simulink subsystem "PvtSubSys_PLAN_DPC"  (R2020b)
settings: Solver=VariableStepAuto  StartTime=0.0  StopTime=10.0  RelTol=1e-3
undefined symbols (not defined in the file or in its folder): P_Global_DxvFrontBumper_m, P_Global_DxvRearBumper_m, P_PLAN_DPC_BrkPointDxFactorF1, P_PLAN_DPC_BrkPointDxFactorF2, P_PLAN_DPC_BrkPointDxFactorF3, P_PLAN_DPC_BrkPointDxFactorF4, P_PLAN_DPC_BrkPointDxFactorR1, P_PLAN_DPC_BrkPointDxFactorR2, P_PLAN_DPC_BrkPointDxFactorR3, P_PLAN_DPC_BrkPointDxFactorR4, P_PLAN_DPC_danqianleida_kaiguan, P_PLAN_DPC_danqianleida_maxDx, P_PLAN_DPC_danqianleida_minDx, P_PLAN_DPC_FrontObj_DX_00, P_PLAN_DPC_FrontObj_DX_03, P_PLAN_DPC_FrontObj_DX_08, P_PLAN_DPC_FrontObj_DX_1, P_PLAN_DPC_HearObj_DX_00, P_PLAN_DPC_HearObj_DX_03, P_PLAN_DPC_HearObj_DX_08, P_PLAN_DPC_HearObj_DX_11, P_PLAN_DPC_HWALineRearA2Factor, P_PLAN_DPC_HWALineRearA3Factor, P_PLAN_DPC_ObjAxLPalpha, P_PLAN_DPC_ObjDxLPalpha, P_PLAN_DPC_ObjDyLPalpha, P_PLAN_DPC_ObjVxLPalpha, P_PLAN_DPC_xiangduisudu_kmh
libraries: simulink x22
(part 3 of 3)

== matlab function PvtSubSys_PLAN_DPC/DPCLock/BufRelease1 ==
  data: LaneChange input; DxvFrontBumper_m input; DxvRearBumper_m input; DPCLe input; DPCRi input; LostBufID input; LostBufRemoveMark output uint8; LostBufDx input; LostBufDy input; LostBufVx input; LostBufDPCLe input; LostBufDPCRi input; LostBufLostAge input; ObjID input; ObjDx input; ObjDy input; ObjVx input; LostBufBreakLockObjID output; LostBufBreakLockCond output; ToleranceBoxFront output; ToleranceBoxRear output; ToleranceBoxLeft output; ToleranceBoxRight output; Obj_Fus_Type input
function [LostBufRemoveMark,LostBufBreakLockObjID,LostBufBreakLockCond,ToleranceBoxFront,ToleranceBoxRear,ToleranceBoxLeft,ToleranceBoxRight]  = LostBufOut(LaneChange, DxvFrontBumper_m,DxvRearBumper_m,DPCLe,DPCRi,LostBufID,LostBufDx,LostBufDy,LostBufVx,LostBufDPCLe,LostBufDPCRi,LostBufLostAge,ObjID,ObjDx, ObjDy, ObjVx, Obj_Fus_Type)

LostBufRemoveMark=uint8(zeros(11,1));%从缓存中移除标志位
LostBufBreakLockObjID=uint8(zeros(11,1));
LostBufBreakLockCond=uint8(zeros(11,1));
ToleranceBoxFront=single(zeros(11,1));
ToleranceBoxRear=single(zeros(11,1));
ToleranceBoxLeft=single(zeros(11,1));
ToleranceBoxRight=single(zeros(11,1));

RadarUnstableZoneX=single(7);

VehCenterX=0.5*(DxvFrontBumper_m-DxvRearBumper_m);
%
for ObjIndex1 =1:11
    if LostBufID(ObjIndex1)~=uint8(0)
        MaxLocktime=max(LostBufDPCLe(ObjIndex1),LostBufDPCRi(ObjIndex1))*8;
        if  LostBufLostAge(ObjIndex1)*0.02 > MaxLocktime %如果超过锁止时间则强制释放
            LostBufRemoveMark(ObjIndex1)=uint8(1);
            LostBufBreakLockCond(ObjIndex1)=uint8(1);
            continue;
        end
        %后续可能需要根据不同位置调整公差带
        if LostBufVx(ObjIndex1)>=0
            ToleranceBoxFrontOffset=3+max(0.02*LostBufLostAge(ObjIndex1),0);%每隔1s多加一米
            ToleranceBoxRearOffset=single(3)+max(0.02*min(LostBufLostAge(ObjIndex1),100)*LostBufVx(ObjIndex1),0);%前1秒不动
            ToleranceBoxLeftOffset=single(1.8)+min(0.02*LostBufLostAge(ObjIndex1),0.8);
            ToleranceBoxRightOffset=single(1.8)+min(0.02*LostBufLostAge(ObjIndex1),0.8);
        else
            ToleranceBoxFrontOffset=single(3)+max(0.02*min(LostBufLostAge(ObjIndex1),100)*LostBufVx(ObjIndex1),0);%前1秒
            ToleranceBoxRearOffset=3+max(0.02*LostBufLostAge(ObjIndex1),0);%每隔1s加一米
            ToleranceBoxLeftOffset=single(1.8)+min(0.02*LostBufLostAge(ObjIndex1),0.8);
            ToleranceBoxRightOffset=single(1.8)+min(0.02*LostBufLostAge(ObjIndex1),0.8);
        end
        
        PreObjDx = LostBufVx(ObjIndex1)*0.02*LostBufLostAge(ObjIndex1)+LostBufDx(ObjIndex1);
        ToleranceBoxFront(ObjIndex1)=PreObjDx+ToleranceBoxFrontOffset;
        ToleranceBoxRear(ObjIndex1)=PreObjDx-ToleranceBoxRearOffset;
        ToleranceBoxLeft(ObjIndex1)=LostBufDy(ObjIndex1)+ToleranceBoxLeftOffset;
        ToleranceBoxRight(ObjIndex1)=LostBufDy(ObjIndex1)-ToleranceBoxRightOffset;
        
        %雷达不稳定区域的处理
        if ToleranceBoxFront(ObjIndex1)>VehCenterX && ToleranceBoxFront(ObjIndex1)<(DxvFrontBumper_m+RadarUnstableZoneX)
            ToleranceBoxFront(ObjIndex1)=(DxvFrontBumper_m+RadarUnstableZoneX);
        end
        if ToleranceBoxRear(ObjIndex1)>VehCenterX && ToleranceBoxRear(ObjIndex1)<(DxvFrontBumper_m+RadarUnstableZoneX)
            ToleranceBoxRear(ObjIndex1)=VehCenterX;
        end  
        if ToleranceBoxFront(ObjIndex1)>-(DxvRearBumper_m+RadarUnstableZoneX) && ToleranceBoxFront(ObjIndex1)<VehCenterX
            ToleranceBoxFront(ObjIndex1)=VehCenterX;
        end
        if ToleranceBoxRear(ObjIndex1)>-(DxvRearBumper_m+RadarUnstableZoneX) && ToleranceBoxRear(ObjIndex1)<VehCenterX
            ToleranceBoxRear(ObjIndex1)=-(DxvRearBumper_m+RadarUnstableZoneX);
        end
            
        for ObjIndex2 =1:11 
            %如果20帧内重新找到ID则停止锁定
            if ObjID(ObjIndex2)==LostBufID(ObjIndex1) && LostBufLostAge(ObjIndex1)<=20 && Obj_Fus_Type(ObjIndex2) ~= 0
                LostBufRemoveMark(ObjIndex1)=uint8(1);
                LostBufBreakLockObjID(ObjIndex1)=ObjID(ObjIndex2);
                LostBufBreakLockCond(ObjIndex1)=uint8(2);
                break;
            end
            %在预测位置存在一个目标则停止锁定
            if ObjID(ObjIndex2)~= uint8(0) ...
                    && ObjDx(ObjIndex2) <= ToleranceBoxFront(ObjIndex1)...
                    && ObjDx(ObjIndex2) >= ToleranceBoxRear(ObjIndex1)...
                    && ObjDy(ObjIndex2) <= ToleranceBoxLeft(ObjIndex1)...
                    && ObjDy(ObjIndex2) >= ToleranceBoxRight(ObjIndex1) &&  Obj_Fus_Type(ObjIndex2) ~= 0
                LostBufRemoveMark(ObjIndex1)=uint8(1);
                LostBufBreakLockObjID(ObjIndex1)=ObjID(ObjIndex2);
                LostBufBreakLockCond(ObjIndex1)=uint8(3);
                break;
            end
        end
    end

if LaneChange
    LostBufRemoveMark=uint8(ones(11,1));
    LostBufBreakLockCond=uint8(4*ones(11,1));
end
end

== matlab function PvtSubSys_PLAN_DPC/DPCLock/LPF/MATLAB Function ==
  data: Alpha input; ID input; IDK1 input; signal input; result output; resultK1 input single
function result  = LowPassFilter(Alpha,ID,IDK1,signal,resultK1)
result=single(zeros(11,1));
for i=1:11
[IDSurvive,IDoldIndex]=ismember(ID(i),IDK1);
if ID(i)~=uint8(0) && IDSurvive
    result(i) = Alpha*(signal(i) - resultK1(IDoldIndex)) + resultK1(IDoldIndex);
else
    result(i)=signal(i);
end
end

== matlab function PvtSubSys_PLAN_DPC/DPCLock/LPF/MATLAB Function1 ==
  data: Alpha input; ID input; IDK1 input; signal input; result output; resultK1 input single
function result  = LowPassFilter(Alpha,ID,IDK1,signal,resultK1)
result=single(zeros(11,1));
for i=1:11
[IDSurvive,IDoldIndex]=ismember(ID(i),IDK1);
if ID(i)~=uint8(0) && IDSurvive
    result(i) = Alpha*(signal(i) - resultK1(IDoldIndex)) + resultK1(IDoldIndex);
else
    result(i)=signal(i);
end
end

== matlab function PvtSubSys_PLAN_DPC/DPCLock/LPF/MATLAB Function2 ==
  data: Alpha input; ID input; IDK1 input; signal input; result output; resultK1 input single
function result  = LowPassFilter(Alpha,ID,IDK1,signal,resultK1)
result=single(zeros(11,1));
for i=1:11
[IDSurvive,IDoldIndex]=ismember(ID(i),IDK1);
if ID(i)~=uint8(0) && IDSurvive
    result(i) = Alpha*(signal(i) - resultK1(IDoldIndex)) + resultK1(IDoldIndex);
else
    result(i)=signal(i);
end
end

== matlab function PvtSubSys_PLAN_DPC/DPCLock/LPF/MATLAB Function3 ==
  data: LineValid input; LineC3 input; SLObjDy output; LineC2 input; LineC1 input; LineC0 input; LineRange input; ObjDy input; ObjDx input
function SLObjDy=SLdyclc(LineValid,LineC3,LineC2,LineC1,LineC0,LineRange,ObjDy,ObjDx)
SLObjDy=single(zeros(11,1));
for i=1:11
    if  ObjDx(i)>0
        LineC3Factor = single(0);
        LineC2Factor = Interp4(0, 1, LineRange, 1, LineRange+20, 0.7, LineRange+40, 0, ObjDx(i));
        dLineDy = (LineC3Factor * LineC3 * ObjDx(i) * ObjDx(i) * ObjDx(i)) + (LineC2Factor * LineC2 * ObjDx(i) * ObjDx(i)) + (LineC1 * ObjDx(i)) + LineC0;
        SLObjDy(i) = ObjDy(i)-dLineDy;
    else 
        LineC3Factor = single(0);
        LineC2Factor = single(0.2);
        dLineDy = ((LineC3Factor * LineC3 * ObjDx(i) * ObjDx(i) * ObjDx(i)) + (LineC2Factor * LineC2 * ObjDx(i) * ObjDx(i)) + (LineC1 * ObjDx(i)) + LineC0);
        SLObjDy(i) = ObjDy(i)-dLineDy;
    end
end
end
function Out = Interp4(x1,z1,x2,z2,x3,z3,x4,z4,In)  %线性插值
if In<=x1
    Out = single(z1);
elseif (In>x1)&&(In<=x2)
    Out = single(z1+ (In-x1)*(z2-z1)/(x2-x1));
elseif (In>x2)&&(In<=x3)
    Out = single(z2+ (In-x2)*(z3-z2)/(x3-x2));
elseif (In>x3)&&(In<=x4)
    Out = single(z3+ (In-x3)*(z4-z3)/(x4-x3));
else
    Out = single(z4);
end
end

== matlab function PvtSubSys_PLAN_DPC/DPCLock/Lock ==
  data: bufferoverflow output; LostBufRemoveMark input; ObjDPCleK1 input; ObjDPCRiK1 input; ObjID input; ObjIDK1 input; ObjDxK1 input; ObjDyK1 input; ObjVxK1 input; LostBufIDK1 input; LostBufDxK1 input; LostBufDyK1 input; LostBufVxK1 input; LostBufDPCLeK1 input; LostBufDPCRiK1 input; LostBufLostAgeK1 input; LostBufID output uint8; LostBufDx output single; LostBufDy output single; LostBufVx output single; LostBufDPCLe output single; LostBufDPCRi output; LostBufLostAge output single
function [bufferoverflow,LostBufID,LostBufDx,LostBufDy,LostBufVx,LostBufDPCLe,LostBufDPCRi,LostBufLostAge] = TimeCalc(LostBufRemoveMark,ObjDPCleK1,ObjDPCRiK1,ObjID,ObjIDK1,ObjDxK1,ObjDyK1,ObjVxK1,LostBufIDK1,LostBufDxK1,LostBufDyK1,LostBufVxK1,LostBufDPCLeK1,LostBufDPCRiK1,LostBufLostAgeK1)

LostBufID=LostBufIDK1;
LostBufDx=LostBufDxK1;
LostBufDy=LostBufDyK1;
LostBufVx=LostBufVxK1;
LostBufDPCLe=LostBufDPCLeK1;
LostBufDPCRi=LostBufDPCRiK1;
LostBufLostAge=LostBufLostAgeK1;
bufferoverflow=false;

%删除被标记需要释放的元素  //释放目标直接赋予0//
for ObjIndex1=1:11%11个目标
    if LostBufRemoveMark(ObjIndex1)~=uint8(0) %不等于0 说明是1//
        LostBufID(ObjIndex1)=uint8(0);
        LostBufDx(ObjIndex1)=single(0);
        LostBufDy(ObjIndex1)=single(0);
        LostBufVx(ObjIndex1)=single(0);
        LostBufDPCLe(ObjIndex1)=single(0);
        LostBufDPCRi(ObjIndex1)=single(0);
        LostBufLostAge(ObjIndex1)=single(0);
    end
end

% 寻找是否有ID丢失并存入buf
for ObjIndex1=1:11
    if ObjIDK1(ObjIndex1)~=0 %上一周期ID不等于0//
        %寻找过程
        findID=false;
        for ObjIndex2 =1:11
            if ObjID(ObjIndex2)==ObjIDK1(ObjIndex1) %当前时刻的id == 上一时刻的id////
                findID=true;
                break;
            end
        end
        %储存过程
        if ~findID %findID没有找到  那就走这个if 这是丢了//
            MaxLostAge=single(0);
            findbufposition=false;
            bufferoverflow=false;
            oldestbufIndex=11;
            for ObjIndex2 =1:11
                if LostBufLostAge(ObjIndex2)>MaxLostAge %LostBufLostAge这是啥意思//
                    MaxLostAge=LostBufLostAge(ObjIndex2);
                    oldestbufIndex=ObjIndex2;
                end
                if LostBufID(ObjIndex2)==0 %缓存未被使用   %这是什么意思///
                    LostBufID(ObjIndex2)=ObjIDK1(ObjIndex1);
                    LostBufDx(ObjIndex2)=ObjDxK1(ObjIndex1);
                    LostBufDy(ObjIndex2)=ObjDyK1(ObjIndex1);
                    LostBufVx(ObjIndex2)=ObjVxK1(ObjIndex1);
                    LostBufDPCLe(ObjIndex2)=ObjDPCleK1(ObjIndex1);
                    LostBufDPCRi(ObjIndex2)=ObjDPCRiK1(ObjIndex1);
                    findbufposition=true;
                    break;
                end
            end
            if ~findbufposition
                LostBufID(oldestbufIndex)=ObjIDK1(ObjIndex1);
                LostBufDx(oldestbufIndex)=ObjDxK1(ObjIndex1);
                LostBufDy(oldestbufIndex)=ObjDyK1(ObjIndex1);
                LostBufVx(oldestbufIndex)=ObjVxK1(ObjIndex1);
                LostBufDPCLe(oldestbufIndex)=ObjDPCleK1(ObjIndex1);
                LostBufDPCRi(oldestbufIndex)=ObjDPCRiK1(ObjIndex1);
                bufferoverflow=true;
            end
            
        end
    end
end

%计算丢失的周期，从1开始
for ObjIndex1 =1:11
    if LostBufID(ObjIndex1)~=uint8(0)
        LostBufLostAge(ObjIndex1)=min(LostBufLostAge(ObjIndex1)+1,500);%LostBufLostAge记录目标丢的时间///
    end
end

%坐标旋转
% for ObjIndex1 =1:11
%     LostBufDx(ObjIndex1) = (LostBufDx(ObjIndex1)-EgoDDeltaX)*EgoCosOfPsi + (LostBufDy(ObjIndex1)-EgoDDeltaY)*EgoSinOfPsi;
%     LostBufDy(ObjIndex1) = -(LostBufDx(ObjIndex1)-EgoDDeltaX)*EgoSinOfPsi + (LostBufDy(ObjIndex1)-EgoDDeltaY)*EgoCosOfPsi;
% end
end

== matlab function PvtSubSys_PLAN_DPC/DPCLock/Release ==
  data: DPCLe input; DPCRi input; LostBufID input; LostBufRemoveMark output uint8; LostBufDx input; LostBufDy input; LostBufVx input; LostBufDPCLe input; LostBufDPCRi input; LostBufLostAge input; ObjID input; ObjDx input; ObjDy input; ObjVx input
function LostBufRemoveMark  = fcn(DPCLe,DPCRi,LostBufID,LostBufDx,LostBufDy,LostBufVx,LostBufDPCLe,LostBufDPCRi,LostBufLostAge,ObjID,ObjDx, ObjDy, ObjVx )

LostBufRemoveMark=uint8(zeros(11,1));
FrontLine1=8;%前向角雷达属性不稳定限制线
RearLine1=-6;%后向角雷达属性不稳定限制线
PreDxOffSet=5;%允许的预测误差

for ObjIndex1 =1:11 %如果超过锁止时间则强制释放
    if LostBufID(ObjIndex1)~=0
        Locktime=max(LostBufDPCLe(ObjIndex1),LostBufDPCRi(ObjIndex1))*10;
        if  LostBufLostAge(ObjIndex1)>Locktime
            LostBufRemoveMark(ObjIndex1)=uint8(1);
        end
    end
end
for ObjIndex1 =1:11
    if LostBufID(ObjIndex1)~=0
        for ObjIndex2 =1:11 %如果十个周期内重新找到ID则停止锁定
            PreObjDx = LostBufVx(ObjIndex1)*LostBufLostAge(ObjIndex1)+LostBufDx(ObjIndex1);
            if ObjID(ObjIndex2)==LostBufID(ObjIndex1) && LostBufLostAge(ObjIndex1)<=10
                LostBufRemoveMark(ObjIndex1)=uint8(1);
                break;
            end
            if LostBufDy(ObjIndex1) > 0 && abs(ObjDx(ObjIndex2)-PreObjDx) < PreDxOffSet && ObjDy(ObjIndex2) > 0  && ObjID(ObjIndex2)~=0 %分两边 如果预测位置有目标则解除锁定
                LostBufRemoveMark(ObjIndex1)=uint8(1);
                break;
            end
            if LostBufDy(ObjIndex1) <= 0 && abs(ObjDx(ObjIndex2)-PreObjDx) < PreDxOffSet && ObjDy(ObjIndex2) <= 0  && ObjID(ObjIndex2)~=0 %分两边 如果预测位置有目标则解除锁定
                LostBufRemoveMark(ObjIndex1)=uint8(1);
                break;
            end
            if PreObjDx<FrontLine1 && PreObjDx>RearLine1 && LostBufDy(ObjIndex1) > 0 && ObjDx(ObjIndex2)<FrontLine1 && ObjDx(ObjIndex2)>RearLine1 && ObjDy(ObjIndex2) > 0 && ObjID(ObjIndex2)~=0  %分两边 前后雷达不可信属性区域内消失的目标,特殊处理一下
                LostBufRemoveMark(ObjIndex1)=uint8(1);
                break;
            end
            if PreObjDx<FrontLine1 && PreObjDx>RearLine1 && LostBufDy(ObjIndex1) <= 0 && ObjDx(ObjIndex2)<FrontLine1 && ObjDx(ObjIndex2)>RearLine1 && ObjDy(ObjIndex2) <= 0 && ObjID(ObjIndex2)~=0  %分两边 前后雷达不可信属性区域内消失的目标,特殊处理一下
                LostBufRemoveMark(ObjIndex1)=uint8(1);
                break;             
            end
            if LostBufDx(ObjIndex1)<FrontLine1 && LostBufDx(ObjIndex1)>RearLine1 && LostBufDy(ObjIndex1) > 0 && ObjDx(ObjIndex2)<FrontLine1 && ObjDx(ObjIndex2)>RearLine1 && ObjDy(ObjIndex2) > 0 && ObjID(ObjIndex2)~=0  %分两边 预测会进入该不可信区域的目标特殊处理一下
                LostBufRemoveMark(ObjIndex1)=uint8(1);
                break;
            end
            if LostBufDx(ObjIndex1)<FrontLine1 && LostBufDx(ObjIndex1)>RearLine1 && LostBufDy(ObjIndex1) <= 0 && ObjDx(ObjIndex2)<FrontLine1 && ObjDx(ObjIndex2)>RearLine1 && ObjDy(ObjIndex2) <= 0 && ObjID(ObjIndex2)~=0  %分两边 预测会进入该不可信区域的目标特殊处理一下
                LostBufRemoveMark(ObjIndex1)=uint8(1);
                break;             
            end
        end
    end
end

== matlab function PvtSubSys_PLAN_DPC/DPCLock/Release1 ==
  data: DPCLe input; DPCRi input; LostBufID input; LostBufRemoveMark output uint8; LostBufDx input; LostBufDy input; LostBufVx input; LostBufDPCLe input; LostBufDPCRi input; LostBufLostAge input; ObjID input; ObjDx input; ObjDy input; ObjVx input
function LostBufRemoveMark  = fcn(DPCLe,DPCRi,LostBufID,LostBufDx,LostBufDy,LostBufVx,LostBufDPCLe,LostBufDPCRi,LostBufLostAge,ObjID,ObjDx, ObjDy, ObjVx )

LostBufRemoveMark=uint8(zeros(11,1));
FrontLine1=8;%前向角雷达属性不稳定限制线
RearLine1=-6;%后向角雷达属性不稳定限制线
PreDxOffSet=5;%允许的预测误差

for ObjIndex1 =1:11 %如果超过锁止时间则强制释放
    if LostBufID(ObjIndex1)~=0
        Locktime=max(LostBufDPCLe(ObjIndex1),LostBufDPCRi(ObjIndex1))*10;
        if  LostBufLostAge(ObjIndex1)>Locktime
            LostBufRemoveMark(ObjIndex1)=uint8(1);
        end
    end
end
for ObjIndex1 =1:11 
    if LostBufID(ObjIndex1)~=0
        PreObjDx = LostBufVx(ObjIndex1)*LostBufLostAge(ObjIndex1)+LostBufDx(ObjIndex1);
        for ObjIndex2 =1:11 %如果十个周期内重新找到ID则停止锁定
            if ObjID(ObjIndex2)==LostBufID(ObjIndex1) && LostBufLostAge(ObjIndex1)<=10
                LostBufRemoveMark(ObjIndex1)=uint8(1);
                break;
            end
        end
        if LostBufDy(ObjIndex1) > 0 %分两边 如果预测位置有目标则解除锁定
            for ObjIndex2 =1:11
                if abs(ObjDx(ObjIndex2)-PreObjDx) < PreDxOffSet && ObjDy(ObjIndex2) > 0  && ObjID(ObjIndex2)~=0
                    LostBufRemoveMark(ObjIndex1)=uint8(1);
                    break;
                end
            end
        end
        if LostBufDy(ObjIndex1) <= 0  %分两边 如果预测位置有目标则解除锁定
            for ObjIndex2 =1:11
                if abs(ObjDx(ObjIndex2)-PreObjDx) < PreDxOffSet && ObjDy(ObjIndex2) <= 0  && ObjID(ObjIndex2)~=0
                    LostBufRemoveMark(ObjIndex1)=uint8(1);
                    break;
                end
            end
        end
        if (LostBufDx(ObjIndex1)<FrontLine1 || PreObjDx<FrontLine1) && (LostBufDx(ObjIndex1)>RearLine1 || PreObjDx>RearLine1) && LostBufDy(ObjIndex1) < 0   %分两边 前后雷达不可信属性区域内消失的目标特殊处理一下
            for ObjIndex2 =1:11
                if ObjDx(ObjIndex2)<FrontLine1 && ObjDx(ObjIndex2)>RearLine1 && ObjDy(ObjIndex2) < 0 && ObjID(ObjIndex2)~=0
                    LostBufRemoveMark(ObjIndex1)=uint8(1);
                    break;
                end
            end
        end
        if (LostBufDx(ObjIndex1)<FrontLine1 || PreObjDx<FrontLine1) && (LostBufDx(ObjIndex1)>RearLine1 || PreObjDx>RearLine1) && LostBufDy(ObjIndex1) > 0 
            for ObjIndex2 =1:11
                if ObjDx(ObjIndex2)<FrontLine1 && ObjDx(ObjIndex2)>RearLine1 && ObjDy(ObjIndex2) > 0 && ObjID(ObjIndex2)~=0
                    LostBufRemoveMark(ObjIndex1)=uint8(1);
                    break;
                end
            end
        end      
    end
end

== matlab function PvtSubSys_PLAN_DPC/DangerPlausCalc/DangerPlaus_Calculate_Radar ==
  data: ObjID input; ObjTimeAlive input; ObjDx input; ObjDxRelCal_FL output; ObjDxRelCal_FR output; ObjDxRelCal_RL output; ObjDxRelCal_RR output; ObjDy input; ObjVx input; Object_Fus_Type input; Object_MovingState input; ESSLineLA3 input; ESSLineLA2 input; ESSLineLA1 input; ESSLineLA0 input; ESSLineLRange input; ESSLineRA3 input; ESSLineRA2 input; ESSLineRA1 input; ESSLineRA0 input; ESSLineRRange input; VehicleSpd_kph input; RoadWidth input; Y_Factor_L output; Y_Factor_R output; L_Oncoming_flag output; R_Oncoming_flag output; NearestObjValid_L output boolean; NearestObjValid_R output boolean; NearestObjSpeed_L output; NearestObjSpeed_R output; ObjVxGnd_1 output; ObjDxRelFinal_FL_1 output; P_VSM_DPC_HWALineRearA2Factor input; P_VSM_DPC_HWALineRearA3Factor input; P_Global_DxvFrontBumper_m input; P_Global_DxvRearBumper_m input
function [ObjDxRelCal_FL,ObjDxRelCal_FR,ObjDxRelCal_RL,ObjDxRelCal_RR,Y_Factor_L,Y_Factor_R,...
    L_Oncoming_flag,R_Oncoming_flag,...
    NearestObjValid_L,NearestObjValid_R,NearestObjSpeed_L,NearestObjSpeed_R, ObjVxGnd_1, ObjDxRelFinal_FL_1] = ...
    fcn(ObjID, ObjTimeAlive, ObjDx, ObjDy, ObjVx, Object_Fus_Type, Object_MovingState,...
    ESSLineLA3, ESSLineLA2,ESSLineLA1, ESSLineLA0, ESSLineLRange,...
    ESSLineRA3, ESSLineRA2,ESSLineRA1, ESSLineRA0, ESSLineRRange,...
    VehicleSpd_kph,RoadWidth,...
    P_VSM_DPC_HWALineRearA2Factor,...
P_VSM_DPC_HWALineRearA3Factor, P_Global_DxvFrontBumper_m, P_Global_DxvRearBumper_m)

InvalidValue = single(999);
ObjTimeAliveCounter = 3;
TimeTurn = 4;
TimeReact = 3;
ObjDxRelCal_FL = zeros(11,1);
ObjDxRelCal_FR = zeros(11,1);
ObjDxRelCal_RL = zeros(11,1);
ObjDxRelCal_RR = zeros(11,1);
DeltaDistance_Y_L = zeros(11,1);
DeltaDistance_Y_R = zeros(11,1);
Y_Factor_L = zeros(11,1);
Y_Factor_R = zeros(11,1);
L_Oncoming = zeros(11,1);
R_Oncoming = zeros(11,1);
VehicleSpd_ms = VehicleSpd_kph / 3.6;

TimePredict_L = (abs(ESSLineLA0) / RoadWidth * TimeTurn) + TimeReact;
TimePredict_R = (abs(ESSLineRA0) / RoadWidth * TimeTurn) + TimeReact;

NearestObjValid_L = false;
NearestObjDx_L = InvalidValue;
NearestObjSpeed_L = InvalidValue;
NearestObjValid_R = false;
NearestObjDx_R = InvalidValue;
NearestObjSpeed_R = InvalidValue;

ObjVxGnd_1 = single(0);
ObjDxRelFinal_FL_1 = single(0);

for i = 1:11
    if (ObjID(i) > 0)...
            && (ObjTimeAlive(i) > ObjTimeAliveCounter)
        ObjVxGnd = ObjVx(i) + VehicleSpd_ms;
        if i == 1   %%%TEST
            ObjVxGnd_1 = ObjVxGnd;
        end
        if ObjDx(i) >= 0   %Front
            ObjDxRelCal_RL(i) = - InvalidValue;
            ObjDxRelCal_RR(i) = - InvalidValue;
            %%%X Calculate%%%
            ObjDxRelInitial_Front = ObjDx(i) - P_Global_DxvFrontBumper_m;
            ObjDxRelFinal_FL = ObjDxRelInitial_Front + (ObjVxGnd * TimePredict_L) - (VehicleSpd_ms * TimePredict_L);
            if i == 1   %%%TEST
                ObjDxRelFinal_FL_1 = ObjDxRelFinal_FL;
            end
            ObjDxRelFinal_FR = ObjDxRelInitial_Front + (ObjVxGnd * TimePredict_R) - (VehicleSpd_ms * TimePredict_R);
            if (ObjDxRelInitial_Front*ObjDxRelFinal_FL)<0   %Very Dangerous
                ObjDxRelCal_FL(i) = 0;
            else
                ObjDxRelCal_FL(i) = min(ObjDxRelInitial_Front,ObjDxRelFinal_FL);
            end
            if (ObjDxRelInitial_Front*ObjDxRelFinal_FR)<0
                ObjDxRelCal_FR(i) = 0;
            else
                ObjDxRelCal_FR(i) = min(ObjDxRelInitial_Front,ObjDxRelFinal_FR);
            end
            %%%Y Calculate%%%
            P_HWALineLFrontA3Factor = single(0);
            P_HWALineRFrontA3Factor = single(0);
            P_HWALineLFrontA2Factor = Interpol(0, 1, ESSLineLRange, 1, ESSLineLRange+20, 0.7, ESSLineLRange+40, 0, ObjDx(i));
            P_HWALineRFrontA2Factor = Interpol(0, 1, ESSLineRRange, 1, ESSLineRRange+20, 0.7, ESSLineRRange+40, 0, ObjDx(i));
            Y_L = (P_HWALineLFrontA3Factor * ESSLineLA3 * ObjDx(i) * ObjDx(i) * ObjDx(i)) + (P_HWALineLFrontA2Factor * ESSLineLA2 * ObjDx(i) * ObjDx(i)) + (ESSLineLA1 * ObjDx(i)) + ESSLineLA0;
            Y_R = (P_HWALineRFrontA3Factor * ESSLineRA3 * ObjDx(i) * ObjDx(i) * ObjDx(i)) + (P_HWALineRFrontA2Factor * ESSLineRA2 * ObjDx(i) * ObjDx(i)) + (ESSLineRA1 * ObjDx(i)) + ESSLineRA0;
            %%%SD%%%
            DeltaDistance_Y_L(i) = abs(ObjDy(i) - Y_L);
            DeltaDistance_Y_R(i) = abs(ObjDy(i) - Y_R);
            %%%Feature Of Nearest Obj Of Next Lane%%%
            if (ObjDy(i) >= (Y_L - (RoadWidth / 2))) && (ObjDy(i) <= (Y_L + (RoadWidth / 2))) && (ObjDx(i) <= NearestObjDx_L)
                NearestObjValid_L = true;
                NearestObjDx_L = ObjDx(i);
                NearestObjSpeed_L = ObjVxGnd;
                if NearestObjSpeed_L < 0
                    L_Oncoming(i) = 1;
                else
                    L_Oncoming(i) = 0;
                end
            elseif (ObjDy(i) >= (Y_R - (RoadWidth / 2))) && (ObjDy(i) <= (Y_R + (RoadWidth / 2))) && (ObjDx(i) <= NearestObjDx_R)
                NearestObjValid_R = true;
                NearestObjDx_R = ObjDx(i);
                NearestObjSpeed_R = ObjVxGnd;
                if NearestObjSpeed_R < 0
                    R_Oncoming(i) = 1;
                else
                    R_Oncoming(i) = 0;
                end
            end
        else   %Rear
            ObjDxRelCal_FL(i) = InvalidValue;
            ObjDxRelCal_FR(i) = InvalidValue;
            %%%X Calculate%%%
            ObjDxRelInitial_Rear = ObjDx(i) + P_Global_DxvRearBumper_m;
            ObjDxRelFinal_RL = ObjDxRelInitial_Rear + (ObjVxGnd * TimePredict_L) - (VehicleSpd_ms * TimePredict_L);
            ObjDxRelFinal_RR = ObjDxRelInitial_Rear + (ObjVxGnd * TimePredict_R) - (VehicleSpd_ms * TimePredict_R);
            if (ObjDxRelInitial_Rear*ObjDxRelFinal_RL)<0
                ObjDxRelCal_RL(i) = 0;
            else
                ObjDxRelCal_RL(i) = max(ObjDxRelInitial_Rear,ObjDxRelFinal_RL);
            end
            
            if (ObjDxRelInitial_Rear*ObjDxRelFinal_RR)<0
                ObjDxRelCal_RR(i) = 0;
            else
                ObjDxRelCal_RR(i) = max(ObjDxRelInitial_Rear,ObjDxRelFinal_RR);
            end
            %%%Y Calculate%%%
            Y_L = (P_VSM_DPC_HWALineRearA3Factor * ESSLineLA3 * ObjDx(i) * ObjDx(i) * ObjDx(i)) + (P_VSM_DPC_HWALineRearA2Factor * ESSLineLA2 * ObjDx(i) * ObjDx(i)) + (ESSLineLA1 * ObjDx(i)) + ESSLineLA0;
            Y_R = (P_VSM_DPC_HWALineRearA3Factor * ESSLineRA3 * ObjDx(i) * ObjDx(i) * ObjDx(i)) + (P_VSM_DPC_HWALineRearA2Factor * ESSLineRA2 * ObjDx(i) * ObjDx(i)) + (ESSLineRA1 * ObjDx(i)) + ESSLineRA0;
            %%%SD%%%
            DeltaDistance_Y_L(i) = abs(ObjDy(i) - Y_L);
            DeltaDistance_Y_R(i) = abs(ObjDy(i) - Y_R);
        end
    else
        ObjDxRelCal_FL(i) = InvalidValue;
        ObjDxRelCal_FR(i) = InvalidValue;
        ObjDxRelCal_RL(i) = - InvalidValue;
        ObjDxRelCal_RR(i) = - InvalidValue;
        DeltaDistance_Y_L(i) = InvalidValue;
        DeltaDistance_Y_R(i) = InvalidValue;
    end
    if (Object_Fus_Type(i) == 0x2) && (Object_MovingState(i) == 0x3)   %F&&Stationary
        Y_Factor_L(i) = Interpol(0, 1, 0.3*RoadWidth, 1, 0.6*RoadWidth, 0, 0.6*RoadWidth+1, 0, DeltaDistance_Y_L(i));
        Y_Factor_R(i) = Interpol(0, 1, 0.3*RoadWidth, 1, 0.6*RoadWidth, 0, 0.6*RoadWidth+1, 0, DeltaDistance_Y_R(i));
    else
        Y_Factor_L(i) = Interpol(0, 1, 0.5*RoadWidth, 1, 0.5*RoadWidth+1, 0, 0.5*RoadWidth+2, 0, DeltaDistance_Y_L(i));
        Y_Factor_R(i) = Interpol(0, 1, 0.5*RoadWidth, 1, 0.5*RoadWidth+1, 0, 0.5*RoadWidth+2, 0, DeltaDistance_Y_R(i));
    end
    L_Oncoming_flag = ismember(1,L_Oncoming);
    R_Oncoming_flag = ismember(1,R_Oncoming);
end

function Out = Interpol(x1,z1,x2,z2,x3,z3,x4,z4,In)
if In<=x1
    Out = single(z1);
elseif (In>x1)&&(In<=x2)
    Out = single(z1+ (In-x1)*(z2-z1)/(x2-x1));
elseif (In>x2)&&(In<=x3)
    Out = single(z2+ (In-x2)*(z3-z2)/(x3-x2));
elseif (In>x3)&&(In<=x4)
    Out = single(z3+ (In-x3)*(z4-z3)/(x4-x3));
else
    Out = single(z4);
end

== matlab function PvtSubSys_PLAN_DPC/DangerPlausCalc3/DangerFactorMatrixCalc_Left ==
  data: VehSpd input; ObjValid input; ObjDx input; ObjDy input; ObjVx input; LineValid input; LineC3 input; LineC2 input; LineC1 input; LineC0 input; LineRange input; LineRearC2Factor input; LineRearC3Factor input; RoadWidth input; MaxObjNum input; obj_front_Dx output; obj_front_Vx output size=[1 11]; obj_Rear_Dx output; obj_Rear_Vx output; PreDyRel output size=[11]; Oncoming_flag output; NearestObjValid output; NearestObjDx output; NearestObjSpeed output; Rear_NearesObjValid output; Rear_NearestObjDx output; Rear_NearestObjSpeed output
function [obj_front_Dx,obj_front_Vx,obj_Rear_Dx,obj_Rear_Vx,PreDyRel,Oncoming_flag,NearestObjValid,NearestObjDx,NearestObjSpeed,Rear_NearesObjValid,Rear_NearestObjDx,Rear_NearestObjSpeed] = ...
    fcn(VehSpd,ObjValid,ObjDx, ObjDy, ObjVx, ...
    LineValid, LineC3, LineC2,LineC1, LineC0, LineRange,...
    LineRearC2Factor,LineRearC3Factor,RoadWidth,MaxObjNum)
% #define
fInvalidValue = single(999);%无效值

%init

PreDyRel = ones(11,1).*fInvalidValue;

NearestObjValid = false;
NearestObjDx = fInvalidValue;
NearestObjSpeed = fInvalidValue;
%/////
Rear_NearesObjValid = false;
Rear_NearestObjDx = -fInvalidValue;
Rear_NearestObjSpeed = -fInvalidValue;
%/////
NearestObj_Oncoming = zeros(11,1);

DxvFrontBumper_m = single(3.8);

DxvRearBumper_m = single(0.9);
RtVehSpdms=VehSpd/3.6;





%新接口信号
Front_fInvalidValue = single(999);%无效值
Rear_fInvalidValue = single(-999);%无效值
obj_front_Dx = ones(1,11).* Front_fInvalidValue;
obj_front_Vx = single(zeros(1,11));
obj_Rear_Dx = ones(1,11).* Rear_fInvalidValue;
obj_Rear_Vx = single(zeros(1,11));



%ObjVx 单位是m/s  /////////

if LineValid ~= 0
    for i = 1:MaxObjNum
        if ObjValid(i) 
                if ObjDx(i) >= 0 %前方目标
                  obj_front_Dx(i) = ObjDx(i);%-0.2-DxvFrontBumper_m;
                  obj_front_Vx(i) = single(ObjVx(i)*3.6+0.5);%m/s转换成km/h  ////////////    
                else %后方目标
                    % dPreCollisionDist = ObjDx(i) + DxvRearBumper_m;%障碍物到车屁股的距离//负值
                  obj_Rear_Dx(i) = ObjDx(i);%-0.2+ DxvRearBumper_m;
                  obj_Rear_Vx(i) = single(ObjVx(i)*3.6+0.5);%m/s转换成km/h  //////////// 
                end
        else
            %do nothing
        end
        %计算横向相对距离和前方目标属性
        if ObjDx(i) >= 0 %前方目标
            LineC3Factor = single(0);
            LineC2Factor = Interp4(0, 1, LineRange, 1, LineRange+20, 0.7, LineRange+40, 0, ObjDx(i));
            dLineDy=(LineC3Factor * LineC3 * ObjDx(i) * ObjDx(i) * ObjDx(i)) + (LineC2Factor * LineC2 * ObjDx(i) * ObjDx(i)) + (LineC1 * ObjDx(i)) + LineC0;
            PreDyRel(i) = ObjDy(i)-dLineDy;
            %前方最近目标属性
            if (ObjDy(i) >= (dLineDy - (RoadWidth / 2))) && (ObjDy(i) <= (dLineDy + (RoadWidth / 2))) && (ObjDx(i) <= NearestObjDx)
                ObjVx_GND = RtVehSpdms + ObjVx(i);
                NearestObjValid = true;
                NearestObjDx = ObjDx(i);
                NearestObjSpeed = ObjVx_GND;
                if NearestObjSpeed < -2.5
                    NearestObj_Oncoming(i) = 1;
                    
                else
                    NearestObj_Oncoming(i) = 0;
                end
            end
        else %后方目标
            %计算横向相对距离
            LineC3Factor = LineRearC3Factor;
            LineC2Factor = LineRearC2Factor;
            dLineDy = ((LineC3Factor * LineC3 * ObjDx(i) * ObjDx(i) * ObjDx(i)) + (LineC2Factor * LineC2 * ObjDx(i) * ObjDx(i)) + (LineC1 * ObjDx(i)) + LineC0);
            PreDyRel(i) = ObjDy(i)-dLineDy;
            %后方最近目标属性
            if (ObjDy(i) >= (dLineDy - (RoadWidth / 2))) && (ObjDy(i) <= (dLineDy + (RoadWidth / 2))) && (ObjDx(i) >= Rear_NearestObjDx)
               ObjVx_GND = RtVehSpdms + ObjVx(i);
               Rear_NearesObjValid = true;
               Rear_NearestObjDx = ObjDx(i);
               Rear_NearestObjSpeed = ObjVx_GND; %绝对速度//
            end
            
        end
    end
    Oncoming_flag = ismember(1,NearestObj_Oncoming);
    
else
    PreDyRel = single(zeros(11,1));
    Oncoming_flag = false;
    NearestObjValid = false;
    Rear_NearesObjValid = false;
    obj_front_Vx = single(zeros(1,11));
    obj_Rear_Vx = single(zeros(1,11));
    obj_front_Dx = ones(1,11).* Front_fInvalidValue;
    obj_Rear_Dx = ones(1,11).* Rear_fInvalidValue;
    
end

end


function Out = Interp4(x1,z1,x2,z2,x3,z3,x4,z4,In)  %线性插值
if In<=x1
    Out = single(z1);
elseif (In>x1)&&(In<=x2)
    Out = single(z1+ (In-x1)*(z2-z1)/(x2-x1));
elseif (In>x2)&&(In<=x3)
    Out = single(z2+ (In-x2)*(z3-z2)/(x3-x2));
elseif (In>x3)&&(In<=x4)
    Out = single(z3+ (In-x3)*(z4-z3)/(x4-x3));
else
    Out = single(z4);
end
end

== matlab function PvtSubSys_PLAN_DPC/DangerPlausCalc3/DangerFactorMatrixCalc_Left1 ==
  data: VehSpd input; ObjValid input; ObjDx input; ObjDy input; ObjVx input; LineValid input; LineC3 input; LineC2 input; LineC1 input; LineC0 input; LineRange input; LineRearC2Factor input; LineRearC3Factor input; RoadWidth input; MaxObjNum input; obj_front_Dx output; obj_front_Vx output size=[1 11]; obj_Rear_Dx output; obj_Rear_Vx output; PreDyRel output size=[11]; Oncoming_flag output; NearestObjValid output; NearestObjDx output; NearestObjSpeed output; Rear_NearesObjValid output; Rear_NearestObjDx output; Rear_NearestObjSpeed output
function [obj_front_Dx,obj_front_Vx,obj_Rear_Dx,obj_Rear_Vx,PreDyRel,Oncoming_flag,NearestObjValid,NearestObjDx,NearestObjSpeed,Rear_NearesObjValid,Rear_NearestObjDx,Rear_NearestObjSpeed] = ...
    fcn(VehSpd,ObjValid,ObjDx, ObjDy, ObjVx, ...
    LineValid, LineC3, LineC2,LineC1, LineC0, LineRange,...
    LineRearC2Factor,LineRearC3Factor,RoadWidth,MaxObjNum)
% #define
fInvalidValue = single(999);%无效值

%init

PreDyRel = ones(11,1).*fInvalidValue;

NearestObjValid = false;
NearestObjDx = fInvalidValue;
NearestObjSpeed = fInvalidValue;
%/////
Rear_NearesObjValid = false;
Rear_NearestObjDx = -fInvalidValue;
Rear_NearestObjSpeed = -fInvalidValue;
%/////
NearestObj_Oncoming = zeros(11,1);

DxvFrontBumper_m = single(3.8);

DxvRearBumper_m = single(0.9);
RtVehSpdms=VehSpd/3.6;





%新接口信号
Front_fInvalidValue = single(999);%无效值
Rear_fInvalidValue = single(-999);%无效值
obj_front_Dx = ones(1,11).* Front_fInvalidValue;
obj_front_Vx = single(zeros(1,11));
obj_Rear_Dx = ones(1,11).* Rear_fInvalidValue;
obj_Rear_Vx = single(zeros(1,11));



%ObjVx 单位是m/s  /////////

if LineValid ~= 0
    for i = 1:MaxObjNum
        if ObjValid(i) 
                if ObjDx(i) >= 0 %前方目标
                  obj_front_Dx(i) = ObjDx(i);%-0.2-DxvFrontBumper_m;
                  obj_front_Vx(i) = single(ObjVx(i)*3.6+0.5);%m/s转换成km/h  ////////////    
                else %后方目标
                    % dPreCollisionDist = ObjDx(i) + DxvRearBumper_m;%障碍物到车屁股的距离//负值
                  obj_Rear_Dx(i) = ObjDx(i);%-0.2+ DxvRearBumper_m;
                  obj_Rear_Vx(i) = single(ObjVx(i)*3.6+0.5);%m/s转换成km/h  //////////// 
                end
        else
            %do nothing
        end
        %计算横向相对距离和前方目标属性
        if ObjDx(i) >= 0 %前方目标
            LineC3Factor = single(0);
            LineC2Factor = Interp4(0, 1, LineRange, 1, LineRange+20, 0.7, LineRange+40, 0, ObjDx(i));
            dLineDy=(LineC3Factor * LineC3 * ObjDx(i) * ObjDx(i) * ObjDx(i)) + (LineC2Factor * LineC2 * ObjDx(i) * ObjDx(i)) + (LineC1 * ObjDx(i)) + LineC0;
            PreDyRel(i) = ObjDy(i)-dLineDy;
            %前方最近目标属性
            if (ObjDy(i) >= (dLineDy - (RoadWidth / 2))) && (ObjDy(i) <= (dLineDy + (RoadWidth / 2))) && (ObjDx(i) <= NearestObjDx)
                ObjVx_GND = RtVehSpdms + ObjVx(i);
                NearestObjValid = true;
                NearestObjDx = ObjDx(i);
                NearestObjSpeed = ObjVx_GND;
                if NearestObjSpeed < -2.5
                    NearestObj_Oncoming(i) = 1;
                    
                else
                    NearestObj_Oncoming(i) = 0;
                end
            end
        else %后方目标
            %计算横向相对距离
            LineC3Factor = LineRearC3Factor;
            LineC2Factor = LineRearC2Factor;
            dLineDy = ((LineC3Factor * LineC3 * ObjDx(i) * ObjDx(i) * ObjDx(i)) + (LineC2Factor * LineC2 * ObjDx(i) * ObjDx(i)) + (LineC1 * ObjDx(i)) + LineC0);
            PreDyRel(i) = ObjDy(i)-dLineDy;
            %后方最近目标属性
            if (ObjDy(i) >= (dLineDy - (RoadWidth / 2))) && (ObjDy(i) <= (dLineDy + (RoadWidth / 2))) && (ObjDx(i) >= Rear_NearestObjDx)
               ObjVx_GND = RtVehSpdms + ObjVx(i);
               Rear_NearesObjValid = true;
               Rear_NearestObjDx = ObjDx(i);
               Rear_NearestObjSpeed = ObjVx_GND; %绝对速度//
            end
            
        end
    end
    Oncoming_flag = ismember(1,NearestObj_Oncoming);
    
else
    PreDyRel = single(zeros(11,1));
    Oncoming_flag = false;
    NearestObjValid = false;
    Rear_NearesObjValid = false;
    obj_front_Vx = single(zeros(1,11));
    obj_Rear_Vx = single(zeros(1,11));
    obj_front_Dx = ones(1,11).* Front_fInvalidValue;
    obj_Rear_Dx = ones(1,11).* Rear_fInvalidValue;
    
end

end


function Out = Interp4(x1,z1,x2,z2,x3,z3,x4,z4,In)  %线性插值
if In<=x1
    Out = single(z1);
elseif (In>x1)&&(In<=x2)
    Out = single(z1+ (In-x1)*(z2-z1)/(x2-x1));
elseif (In>x2)&&(In<=x3)
    Out = single(z2+ (In-x2)*(z3-z2)/(x3-x2));
elseif (In>x3)&&(In<=x4)
    Out = single(z3+ (In-x3)*(z4-z3)/(x4-x3));
else
    Out = single(z4);
end
end

== matlab function PvtSubSys_PLAN_DPC/DangerPlausCalc3/DangerFactorMatrixCalc_Left2 ==
  data: VehSpd input; ObjValid input; ObjDx input; ObjDy input; ObjVx input; LineValid input; LineC3 input; LineC2 input; LineC1 input; LineC0 input; LineRange input; LineRearC2Factor input; LineRearC3Factor input; RoadWidth input; MaxObjNum input; obj_front_Dx output; obj_front_Vx output size=[1 11]; obj_Rear_Dx output; obj_Rear_Vx output; PreDyRel output size=[11]; Oncoming_flag output; NearestObjValid output; NearestObjDx output; NearestObjSpeed output; Rear_NearesObjValid output; Rear_NearestObjDx output; Rear_NearestObjSpeed output
function [obj_front_Dx,obj_front_Vx,obj_Rear_Dx,obj_Rear_Vx,PreDyRel,Oncoming_flag,NearestObjValid,NearestObjDx,NearestObjSpeed,Rear_NearesObjValid,Rear_NearestObjDx,Rear_NearestObjSpeed] = ...
    fcn(VehSpd,ObjValid,ObjDx, ObjDy, ObjVx, ...
    LineValid, LineC3, LineC2,LineC1, LineC0, LineRange,...
    LineRearC2Factor,LineRearC3Factor,RoadWidth,MaxObjNum)
% #define
fInvalidValue = single(999);%无效值

%init

PreDyRel = ones(11,1).*fInvalidValue;

NearestObjValid = false;
NearestObjDx = fInvalidValue;
NearestObjSpeed = fInvalidValue;
%/////
Rear_NearesObjValid = false;
Rear_NearestObjDx = -fInvalidValue;
Rear_NearestObjSpeed = -fInvalidValue;
%/////
NearestObj_Oncoming = zeros(11,1);

DxvFrontBumper_m = single(3.8);

DxvRearBumper_m = single(0.9);
RtVehSpdms=VehSpd/3.6;





%新接口信号
Front_fInvalidValue = single(999);%无效值
Rear_fInvalidValue = single(-999);%无效值
obj_front_Dx = ones(1,11).* Front_fInvalidValue;
obj_front_Vx = single(zeros(1,11));
obj_Rear_Dx = ones(1,11).* Rear_fInvalidValue;
obj_Rear_Vx = single(zeros(1,11));



%ObjVx 单位是m/s  /////////

if LineValid ~= 0
    for i = 1:MaxObjNum
        if ObjValid(i) 
                if ObjDx(i) >= 0 %前方目标
                  obj_front_Dx(i) = ObjDx(i);%-0.2-DxvFrontBumper_m;
                  obj_front_Vx(i) = single(ObjVx(i)*3.6+0.5);%m/s转换成km/h  ////////////    
                else %后方目标
                    % dPreCollisionDist = ObjDx(i) + DxvRearBumper_m;%障碍物到车屁股的距离//负值
                  obj_Rear_Dx(i) = ObjDx(i);%-0.2+ DxvRearBumper_m;
                  obj_Rear_Vx(i) = single(ObjVx(i)*3.6+0.5);%m/s转换成km/h  //////////// 
                end
        else
            %do nothing
        end
        %计算横向相对距离和前方目标属性
        if ObjDx(i) >= 0 %前方目标
            LineC3Factor = single(0);
            LineC2Factor = Interp4(0, 1, LineRange, 1, LineRange+20, 0.7, LineRange+40, 0, ObjDx(i));
            dLineDy=(LineC3Factor * LineC3 * ObjDx(i) * ObjDx(i) * ObjDx(i)) + (LineC2Factor * LineC2 * ObjDx(i) * ObjDx(i)) + (LineC1 * ObjDx(i)) + LineC0;
            PreDyRel(i) = ObjDy(i)-dLineDy;
            %前方最近目标属性
            if (ObjDy(i) >= (dLineDy - (RoadWidth / 2))) && (ObjDy(i) <= (dLineDy + (RoadWidth / 2))) && (ObjDx(i) <= NearestObjDx)
                ObjVx_GND = RtVehSpdms + ObjVx(i);
                NearestObjValid = true;
                NearestObjDx = ObjDx(i);
                NearestObjSpeed = ObjVx_GND;
                if NearestObjSpeed < -2.5
                    NearestObj_Oncoming(i) = 1;
                    
                else
                    NearestObj_Oncoming(i) = 0;
                end
            end
        else %后方目标
            %计算横向相对距离
            LineC3Factor = LineRearC3Factor;
            LineC2Factor = LineRearC2Factor;
            dLineDy = ((LineC3Factor * LineC3 * ObjDx(i) * ObjDx(i) * ObjDx(i)) + (LineC2Factor * LineC2 * ObjDx(i) * ObjDx(i)) + (LineC1 * ObjDx(i)) + LineC0);
            PreDyRel(i) = ObjDy(i)-dLineDy;
            %后方最近目标属性
            if (ObjDy(i) >= (dLineDy - (RoadWidth / 2))) && (ObjDy(i) <= (dLineDy + (RoadWidth / 2))) && (ObjDx(i) >= Rear_NearestObjDx)
               ObjVx_GND = RtVehSpdms + ObjVx(i);
               Rear_NearesObjValid = true;
               Rear_NearestObjDx = ObjDx(i);
               Rear_NearestObjSpeed = ObjVx_GND; %绝对速度//
            end
            
        end
    end
    Oncoming_flag = ismember(1,NearestObj_Oncoming);
    
else
    PreDyRel = single(zeros(11,1));
    Oncoming_flag = false;
    NearestObjValid = false;
    Rear_NearesObjValid = false;
    obj_front_Vx = single(zeros(1,11));
    obj_Rear_Vx = single(zeros(1,11));
    obj_front_Dx = ones(1,11).* Front_fInvalidValue;
    obj_Rear_Dx = ones(1,11).* Rear_fInvalidValue;
    
end

end


function Out = Interp4(x1,z1,x2,z2,x3,z3,x4,z4,In)  %线性插值
if In<=x1
    Out = single(z1);
elseif (In>x1)&&(In<=x2)
    Out = single(z1+ (In-x1)*(z2-z1)/(x2-x1));
elseif (In>x2)&&(In<=x3)
    Out = single(z2+ (In-x2)*(z3-z2)/(x3-x2));
elseif (In>x3)&&(In<=x4)
    Out = single(z3+ (In-x3)*(z4-z3)/(x4-x3));
else
    Out = single(z4);
end
end

== matlab function PvtSubSys_PLAN_DPC/DangerPlausCalc3/Subsystem/MATLAB Function ==
  data: Object_MovingState input; ObjStationaryFlag output
function ObjStationaryFlag = fcn(Object_MovingState)
ObjStationaryFlag=zeros(11,1);
for i = 1 : 11
    if Object_MovingState(i)==3
        ObjStationaryFlag(i)=1;
    end
end

== matlab function PvtSubSys_PLAN_DPC/DangerPlausCalc3/Subsystem1/MATLAB Function ==
  data: Alpha input; ID input; IDK1 input; signal input; result output; resultK1 input single
function result  = LowPassFilter(Alpha,ID,IDK1,signal,resultK1)
result=single(zeros(11,1));
for i=1:11
[IDSurvive,IDoldIndex]=ismember(ID(i),IDK1);
if ID(i)~=uint8(0) && IDSurvive
    result(i) = Alpha*(signal(i) - resultK1(IDoldIndex)) + resultK1(IDoldIndex);
else
    result(i)=signal(i);
end
end

== matlab function PvtSubSys_PLAN_DPC/DangerPlausCalc3/Subsystem1/MATLAB Function1 ==
  data: Alpha input; ID input; IDK1 input; signal input; result output; resultK1 input single
function result  = LowPassFilter(Alpha,ID,IDK1,signal,resultK1)
result=single(zeros(11,1));
for i=1:11
[IDSurvive,IDoldIndex]=ismember(ID(i),IDK1);
if ID(i)~=uint8(0) && IDSurvive
    result(i) = Alpha*(signal(i) - resultK1(IDoldIndex)) + resultK1(IDoldIndex);
else
    result(i)=signal(i);
end
end

== matlab function PvtSubSys_PLAN_DPC/DangerPlausCalc3/Subsystem1/MATLAB Function2 ==
  data: Alpha input; ID input; IDK1 input; signal input; result output; resultK1 input single
function result  = LowPassFilter(Alpha,ID,IDK1,signal,resultK1)
result=single(zeros(11,1));
for i=1:11
[IDSurvive,IDoldIndex]=ismember(ID(i),IDK1);
if ID(i)~=uint8(0) && IDSurvive
    result(i) = Alpha*(signal(i) - resultK1(IDoldIndex)) + resultK1(IDoldIndex);
else
    result(i)=signal(i);
end
end

== matlab function PvtSubSys_PLAN_DPC/DangerPlausCalc3/Subsystem1/MATLAB Function3 ==
  data: Alpha input; ID input; IDK1 input; signal input; result output; resultK1 input single
function result  = LowPassFilter(Alpha,ID,IDK1,signal,resultK1)
result=single(zeros(11,1));
for i=1:11
[IDSurvive,IDoldIndex]=ismember(ID(i),IDK1);
if ID(i)~=uint8(0) && IDSurvive
    result(i) = Alpha*(signal(i) - resultK1(IDoldIndex)) + resultK1(IDoldIndex);
else
    result(i)=signal(i);
end
end

== matlab function PvtSubSys_PLAN_DPC/Subsystem/RoadWidthCalc ==
  data: LaneExistL1 input; C0L1 input single; C1L1 input single; LaneExistR1 input; C0R1 input; C1R1 input single; RoadWidth output single; RoadWidthK1 input single
function RoadWidth  = VisRoadWidth(LaneExistL1,C0L1,C1L1,LaneExistR1,C0R1,C1R1,RoadWidthK1)

RoadWidth = RoadWidthK1;
Update = false;
temp = single(0);

if (LaneExistL1>1.5)&&(LaneExistR1>1.5)   %%%0x2:Exist
    if abs(57.3*(atan(C1L1) - atan(C1R1)))<3
        temp = (C0L1 - C0R1)/sqrt(C1L1^2 + 1);
        Update = true;
    end
end
if Update
    RoadWidth = 0.1*(temp - RoadWidthK1) + RoadWidthK1;
end
